simulink model "F8_Example_sim"  (R2016a)
settings: Solver=ode15s  StartTime=0.0  StopTime=10  RelTol=1e-4
values from neighbouring files (symbols this model uses):
  umax = 15    [F8_Example.m]
libraries: cstblocks x9
settings Model: Creator=fbianchi  LastModifiedBy=ferna
settings SolverCC: SolverResetMethod=Robust
settings DataIOCC: LimitDataPoints=on  SaveFormat=Array  SignalLoggingSaveFormat=ModelDataLogs
settings OptimizationCC: ExpressionDepthLimit=2147483647  InitFltsAndDblsToZero=on
settings DebuggingCC: AlgebraicLoopMsg=none  SaveWithParameterizedLinksMsg=none  UnderspecifiedInitializationDetection=Classic  MergeDetectMultiDrivingBlocksExec=none  SignalResolutionControl=TryResolveAllWithWarning  SolverPrmCheckMsg=warning  MultiTaskDSMMsg=warning  MultiTaskCondExecSysMsg=none  FcnCallInpInsideContextMsg=UseLocalSettings  StateNameClashWarn=warning
settings HardwareCC: ProdBitPerPointer=32  ProdLargestAtomicFloat=None  ProdIntDivRoundTo=Undefined  ProdEndianess=Unspecified  ProdWordSize=32  ProdHWDeviceType=32-bit Generic
settings ModelReferenceCC: PropagateSignalLabelsOutOfModel=off
settings GRTTargetCC: TargetFcnLib=ansi_tfl_tmw.mat  CombineOutputUpdateFcns=off  GRTInterface=on
settings ConfigComp: CovModelRefEnable=Off

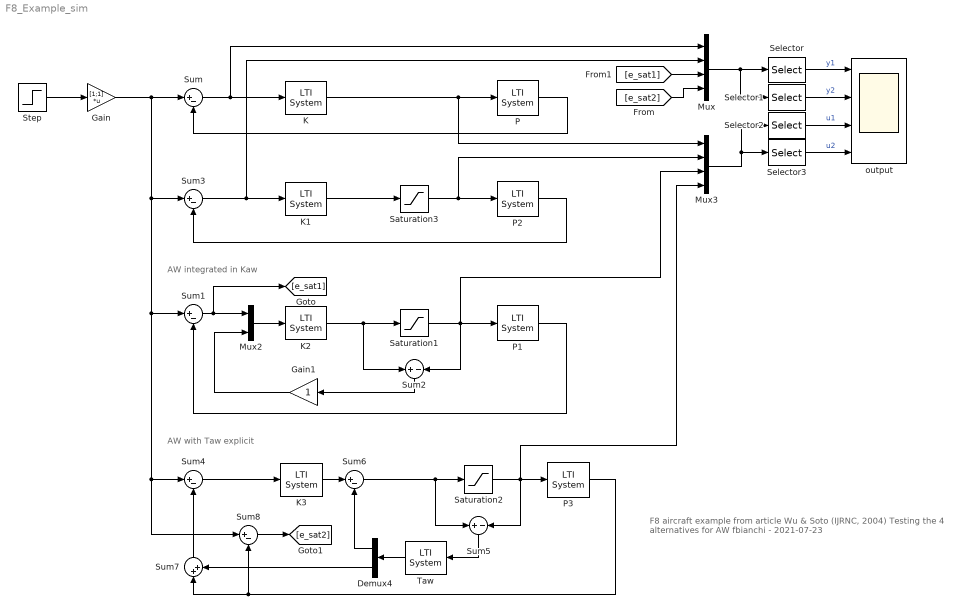
== system F8_Example_sim ==
  note: AW integrated in Kaw
  note: AW with Taw explicit
  note: F8 aircraft example from article Wu & Soto (IJRNC, 2004)
      |
      | Testing the 4 alternatives for AW
      |
      | fbianchi - 2021-07-23
  Demux4 : Demux  Outputs=[2 2]
  Gain : Gain  Gain=[1;1]  Multiplication=Matrix(K*u)
  Gain1 : Gain
  K : cstblocks/LTI System  sys=K  IC=0
  K1 : cstblocks/LTI System  sys=K  IC=0
  K2 : cstblocks/LTI System  sys=Kaw  IC=0
  K3 : cstblocks/LTI System  sys=K  IC=0
  Mux : Mux  Inputs=[2 2 2 2]
  Mux2 : Mux  Inputs=2
  Mux3 : Mux  Inputs=[2 2 2 2]
  P{,1..3} (4 alike) : cstblocks/LTI System  sys=G  IC=0
  Saturation1 : Saturate  UpperLimit=umax  LowerLimit=-umax
  Saturation2 : Saturate  UpperLimit=umax  LowerLimit=-umax
  Saturation3 : Saturate  UpperLimit=umax  LowerLimit=-umax
  Selector : Selector  InputPortWidth=8  IndexOptions=Index vector (dialog)  Indices=[1 3 5 7]  OutputSizes=1
  Selector1 : Selector  InputPortWidth=8  IndexOptions=Index vector (dialog)  Indices=[2 4 6 8]  OutputSizes=1
  Selector2 : Selector  InputPortWidth=8  IndexOptions=Index vector (dialog)  Indices=[1 3 5 7]  OutputSizes=1
  Selector3 : Selector  InputPortWidth=8  IndexOptions=Index vector (dialog)  Indices=[2 4 6 8]  OutputSizes=1
  Step : Step  After=10  SampleTime=0
  Sum{,1,3..4,6,8} (6 alike) : Sum  Inputs=|+-
  Sum2 : Sum  Inputs=+-
  Sum5 : Sum  Inputs=+-
  Sum7 : Sum  Inputs=|++
  Taw : cstblocks/LTI System  sys=Taw  IC=0
  output : Scope  NumInputPorts=4
  wires:
  Sum/1 -> Mux/1, K/1
  P/1 -> Sum/2
  K/1 -> P/1, Mux3/1
  P1/1 -> Sum1/2
  P2/1 -> Sum3/2
  K1/1 -> Saturation3/1
  Saturation3/1 -> Mux3/2, P2/1
  Sum1/1 -> [e_sat1], Mux2/1
  Mux2/1 -> K2/1
  K2/1 -> Saturation1/1, Sum2/1
  Sum3/1 -> Mux/2, K1/1
  Saturation1/1 -> P1/1, Mux3/3, Sum2/2
  Sum2/1 -> Gain1/1
  P3/1 -> Sum8/2, Sum7/1
  Sum4/1 -> K3/1
  Saturation2/1 -> Mux3/4, Sum5/2, P3/1
  Sum5/1 -> Taw/1
  K3/1 -> Sum6/1
  Sum6/1 -> Saturation2/1, Sum5/1
  Taw/1 -> Demux4/1
  Sum7/1 -> Sum4/2
  Mux3/1 -> Selector3/1, Selector2/1
  Gain/1 -> Sum4/1, Sum8/1, Sum1/1, Sum3/1, Sum/1
  Gain1/1 -> Mux2/2
  Mux/1 -> Selector/1, Selector1/1
  Selector/1 -> output/1  "y1"
  Selector1/1 -> output/2  "y2"
  Selector2/1 -> output/3  "u1"
  Selector3/1 -> output/4  "u2"
  Step/1 -> Gain/1
  [e_sat2] -> Mux/4
  [e_sat1] -> Mux/3
  Sum8/1 -> [e_sat2]
  Demux4/1 -> Sum6/2
  Demux4/2 -> Sum7/2
